simulink model "VFA_lin_2015a"  (Simulink 8.5)
settings: Solver=ode45  StartTime=0.0  StopTime=10.0  RelTol=1e-3
undefined symbols (not defined in the file or in its folder): data, stateinit
settings Model: Creator=Travis  LastModifiedBy=ben
settings OptimizationCC: BlockReduction=off  InlineParams=on  BufferReuse=off  InitFltsAndDblsToZero=on
settings DebuggingCC: SaveWithParameterizedLinksMsg=none  SignalResolutionControl=TryResolveAllWithWarning  SolverPrmCheckMsg=warning  MultiTaskDSMMsg=warning  MultiTaskCondExecSysMsg=none  FcnCallInpInsideContextMsg=EnableAllAsWarning  InitInArrayFormatMsg=none  StrictBusMsg=Warning
settings GRTTargetCC: TargetFcnLib=ansi_tfl_tmw.mat

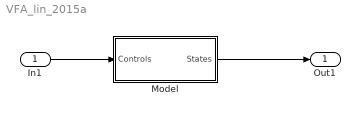
== system VFA_lin_2015a ==
  In1 : Inport
  Model : Subsystem
  Out1 : Outport
  wires:
  Model/1(States) -> Out1/1
  In1/1 -> Model/1(Controls)

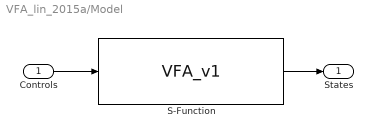
== system VFA_lin_2015a/Model ==
  Controls : Inport
  S-Function : S-Function  FunctionName=VFA_v1  Parameters=data,stateinit  SFunctionDeploymentMode=off  EnableBusSupport=off
  States : Outport
  wires:
  Controls/1 -> S-Function/1
  S-Function/1 -> States/1
